simulink model "buoyEng_th"  (R2022a)
settings: Solver=VariableStepAuto  StartTime=0.0  StopTime=simTime  RelTol=1e-3
values from neighbouring files (symbols this model uses):
  ctrlInput = 10    [buoyEng_ts.m]
  eulAng = [0 0 0]    [buoyEng_ts.m]
libraries: buoyEng_ul x1
settings Model: Creator=mitch  LastModifiedBy=lhill8
settings SolverCC: AlgebraicLoopSolver=TrustRegion
settings DebuggingCC: UnconnectedInputMsg=warning  UnconnectedOutputMsg=warning  UnconnectedLineMsg=warning  SFMachineParentedDataDiag=warning

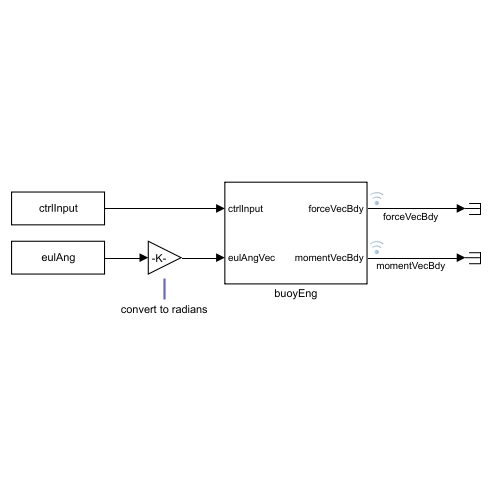
[thumbnail: Simulink's stored preview of the top-level diagram]
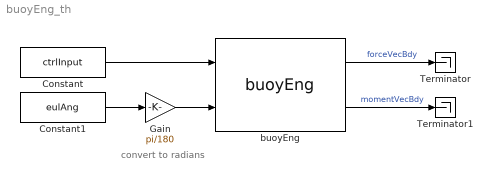
== system buoyEng_th ==
  note: convert to radians
  Constant : Constant  Value=ctrlInput
  Constant1 : Constant  Value=eulAng
  Gain : Gain  Gain=pi/180
  Terminator : Terminator
  Terminator1 : Terminator
  buoyEng : buoyEng_ul/buoyEng  SystemSampleTime=-1  VariantActivationTime=update diagram  Latency=0  AutoFrameSizeCalculation=off
  wires:
  Constant/1 -> buoyEng/1
  Constant1/1 -> Gain/1
  buoyEng/1 -> Terminator/1  "forceVecBdy"
  buoyEng/2 -> Terminator1/1  "momentVecBdy"
  Gain/1 -> buoyEng/2
